simulink model "FDMA"  (Simulink 7.6)
settings: Solver=ode45  StartTime=0.0  StopTime=10.0  RelTol=1e-3
undefined symbols (not defined in the file): get, One, sided
libraries: dsparch4 x6, commanapbnd3 x6, dspsnks4 x6, commchan3 x1
settings Model: Creator=matlab  LastModifiedBy=matlab

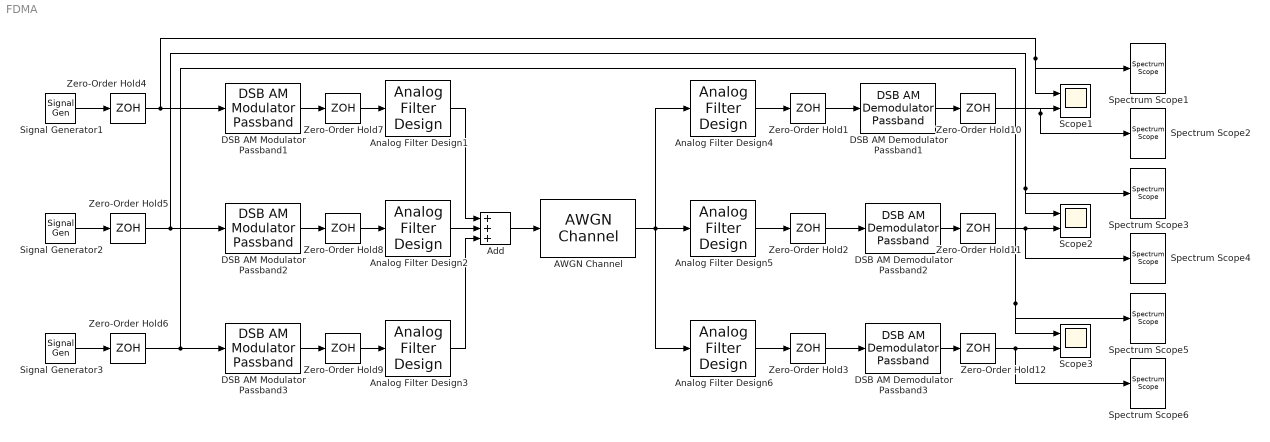
== system FDMA ==
  AWGN Channel : commchan3/AWGN Channel  SystemSampleTime=-1  InputProcessing=Columns as channels (frame based)  seed=67  noiseMode=Variance from mask  EbNodB=10  EsNodB=10  SNRdB=10  bitsPerSym=1  Ps=1  Tsym=1  variance=0.01
  Add : Sum  Inputs=+++
  Analog Filter Design1 : dsparch4/Analog Filter Design  method=Butterworth  filttype=Bandpass  N=8  Wlo=35*2*pi  Whi=45*2*pi  Rp=2  Rs=40
  Analog Filter Design2 : dsparch4/Analog Filter Design  method=Butterworth  filttype=Bandpass  N=8  Wlo=55*2*pi  Whi=65*2*pi  Rp=2  Rs=40
  Analog Filter Design3 : dsparch4/Analog Filter Design  method=Butterworth  filttype=Bandpass  N=8  Wlo=75*2*pi  Whi=85*2*pi  Rp=2  Rs=40
  Analog Filter Design4 : dsparch4/Analog Filter Design  method=Butterworth  filttype=Bandpass  N=8  Wlo=35*2*pi  Whi=45*2*pi  Rp=2  Rs=40
  Analog Filter Design5 : dsparch4/Analog Filter Design  method=Butterworth  filttype=Bandpass  N=8  Wlo=55*2*pi  Whi=65*2*pi  Rp=2  Rs=40
  Analog Filter Design6 : dsparch4/Analog Filter Design  method=Butterworth  filttype=Bandpass  N=8  Wlo=75*2*pi  Whi=85*2*pi  Rp=2  Rs=40
  DSB AM Demodulator Passband1 : commanapbnd3/DSB AM Demodulator Passband  SystemSampleTime=-1  Fc=40  Ph=0  method=Butterworth  n=4  cf=20  Rp=0.1  Rs=50  Offset=1
  DSB AM Demodulator Passband2 : commanapbnd3/DSB AM Demodulator Passband  SystemSampleTime=-1  Fc=60  Ph=0  method=Butterworth  n=4  cf=20  Rp=0.1  Rs=50  Offset=1
  DSB AM Demodulator Passband3 : commanapbnd3/DSB AM Demodulator Passband  SystemSampleTime=-1  Fc=80  Ph=0  method=Butterworth  n=4  cf=20  Rp=0.1  Rs=50  Offset=1
  DSB AM Modulator Passband1 : commanapbnd3/DSB AM Modulator Passband  SystemSampleTime=-1  Fc=40  Ph=0  Offset=1
  DSB AM Modulator Passband2 : commanapbnd3/DSB AM Modulator Passband  SystemSampleTime=-1  Fc=60  Ph=0  Offset=1
  DSB AM Modulator Passband3 : commanapbnd3/DSB AM Modulator Passband  SystemSampleTime=-1  Fc=80  Ph=0  Offset=1
  Scope1 : Scope  NumInputPorts=2
      settings: YMin=-5~-5  YMax=5~5  SampleInput=on  SampleTime=0.01
  Scope2 : Scope  NumInputPorts=2
      settings: YMin=-5~-5  YMax=5~5  SaveName=ScopeData2  SampleInput=on  SampleTime=0.01
  Scope3 : Scope  NumInputPorts=2
      settings: YMin=-5~-5  YMax=5~5  SampleInput=on  SampleTime=0.01
  Signal Generator1 : SignalGenerator  Frequency=4
  Signal Generator2 : SignalGenerator  WaveForm=square  Frequency=0.5
  Signal Generator3 : SignalGenerator  WaveForm=sawtooth
  Spectrum Scope1 : dspsnks4/Spectrum Scope  DialogController=dspdialog.SpectrumScope  DialogControllerArgs=DataTag1  SystemSampleTime=-1  ScopeProperties=on  Domain=Frequency  HorizSpan=1  UseBuffer=on  BufferSize=512  Overlap=256  inpFftLenInherit=on  FFTlength=4096  numAvg=16  DisplayProperties=off  AxisGrid=on  Memory=off  FrameNumber=on  AxisLegend=off  AxisZoom=off  OpenScopeAtSimStart=on  OpenScopeImmediately=off  FigPos=get(0,'defaultfigureposition')  AxisProperties=off  XUnits=Hertz  XRange=One-sided ([0...Fs/2])  XDisplay=0  InheritXIncr=off  XIncr=0.001  XLabel=Samples  XLimit=Auto  YUnits=Watts/Hertz  XMax=1  XMin=0  YLabel=Magnitude-squared, dB  LineProperties=off  wintypeSpecScope=Hann  RsSpecScope=50  betaSpecScope=5  winsampSpecScope=Periodic  XAxisParamsVer=6.9
      settings: YMin=0  YMax=0.40238
  Spectrum Scope2 : dspsnks4/Spectrum Scope  DialogController=dspdialog.SpectrumScope  DialogControllerArgs=DataTag2  SystemSampleTime=-1  ScopeProperties=on  Domain=Frequency  HorizSpan=1  UseBuffer=on  BufferSize=512  Overlap=256  inpFftLenInherit=on  FFTlength=4096  numAvg=16  DisplayProperties=off  AxisGrid=on  Memory=off  FrameNumber=on  AxisLegend=off  AxisZoom=off  OpenScopeAtSimStart=on  OpenScopeImmediately=off  FigPos=get(0,'defaultfigureposition')  AxisProperties=off  XUnits=Hertz  XRange=One-sided ([0...Fs/2])  XDisplay=0  InheritXIncr=off  XIncr=0.001  XLabel=Samples  XLimit=Auto  YUnits=Watts/Hertz  XMax=1  XMin=0  YLabel=Magnitude-squared, dB  LineProperties=off  wintypeSpecScope=Hann  RsSpecScope=50  betaSpecScope=5  winsampSpecScope=Periodic  XAxisParamsVer=6.9
      settings: YMin=0  YMax=0.40238
  Spectrum Scope3 : dspsnks4/Spectrum Scope  DialogController=dspdialog.SpectrumScope  DialogControllerArgs=DataTag3  SystemSampleTime=-1  ScopeProperties=on  Domain=Frequency  HorizSpan=1  UseBuffer=on  BufferSize=512  Overlap=256  inpFftLenInherit=on  FFTlength=4096  numAvg=16  DisplayProperties=off  AxisGrid=on  Memory=off  FrameNumber=on  AxisLegend=off  AxisZoom=off  OpenScopeAtSimStart=on  OpenScopeImmediately=off  FigPos=get(0,'defaultfigureposition')  AxisProperties=off  XUnits=Hertz  XRange=One-sided ([0...Fs/2])  XDisplay=0  InheritXIncr=off  XIncr=0.001  XLabel=Samples  XLimit=Auto  YUnits=Watts/Hertz  XMax=1  XMin=0  YLabel=Magnitude-squared, dB  LineProperties=off  wintypeSpecScope=Hann  RsSpecScope=50  betaSpecScope=5  winsampSpecScope=Periodic  XAxisParamsVer=6.9
      settings: YMin=0  YMax=0.40238
  Spectrum Scope4 : dspsnks4/Spectrum Scope  DialogController=dspdialog.SpectrumScope  DialogControllerArgs=DataTag4  SystemSampleTime=-1  ScopeProperties=on  Domain=Frequency  HorizSpan=1  UseBuffer=on  BufferSize=512  Overlap=256  inpFftLenInherit=on  FFTlength=4096  numAvg=16  DisplayProperties=off  AxisGrid=on  Memory=off  FrameNumber=on  AxisLegend=off  AxisZoom=off  OpenScopeAtSimStart=on  OpenScopeImmediately=off  FigPos=get(0,'defaultfigureposition')  AxisProperties=off  XUnits=Hertz  XRange=One-sided ([0...Fs/2])  XDisplay=0  InheritXIncr=off  XIncr=0.001  XLabel=Samples  XLimit=Auto  YUnits=Watts/Hertz  XMax=1  XMin=0  YLabel=Magnitude-squared, dB  LineProperties=off  wintypeSpecScope=Hann  RsSpecScope=50  betaSpecScope=5  winsampSpecScope=Periodic  XAxisParamsVer=6.9
      settings: YMin=0  YMax=0.40238
  Spectrum Scope5 : dspsnks4/Spectrum Scope  DialogController=dspdialog.SpectrumScope  DialogControllerArgs=DataTag5  SystemSampleTime=-1  ScopeProperties=on  Domain=Frequency  HorizSpan=1  UseBuffer=on  BufferSize=512  Overlap=256  inpFftLenInherit=on  FFTlength=4096  numAvg=16  DisplayProperties=off  AxisGrid=on  Memory=off  FrameNumber=on  AxisLegend=off  AxisZoom=off  OpenScopeAtSimStart=on  OpenScopeImmediately=off  FigPos=get(0,'defaultfigureposition')  AxisProperties=off  XUnits=Hertz  XRange=One-sided ([0...Fs/2])  XDisplay=0  InheritXIncr=off  XIncr=0.001  XLabel=Samples  XLimit=Auto  YUnits=Watts/Hertz  XMax=1  XMin=0  YLabel=Magnitude-squared, dB  LineProperties=off  wintypeSpecScope=Hann  RsSpecScope=50  betaSpecScope=5  winsampSpecScope=Periodic  XAxisParamsVer=6.9
      settings: YMin=0  YMax=0.40238
  Spectrum Scope6 : dspsnks4/Spectrum Scope  DialogController=dspdialog.SpectrumScope  DialogControllerArgs=DataTag6  SystemSampleTime=-1  ScopeProperties=on  Domain=Frequency  HorizSpan=1  UseBuffer=on  BufferSize=512  Overlap=256  inpFftLenInherit=on  FFTlength=4096  numAvg=16  DisplayProperties=off  AxisGrid=on  Memory=off  FrameNumber=on  AxisLegend=off  AxisZoom=off  OpenScopeAtSimStart=on  OpenScopeImmediately=off  FigPos=get(0,'defaultfigureposition')  AxisProperties=off  XUnits=Hertz  XRange=One-sided ([0...Fs/2])  XDisplay=0  InheritXIncr=off  XIncr=0.001  XLabel=Samples  XLimit=Auto  YUnits=Watts/Hertz  XMax=1  XMin=0  YLabel=Magnitude-squared, dB  LineProperties=off  wintypeSpecScope=Hann  RsSpecScope=50  betaSpecScope=5  winsampSpecScope=Periodic  XAxisParamsVer=6.9
      settings: YMin=0  YMax=0.40238
  Zero-Order Hold{1..12} (12 alike) : ZeroOrderHold  SampleTime=0.001
  wires:
  Analog Filter Design2/1 -> Add/2
  Signal Generator1/1 -> Zero-Order Hold4/1
  Signal Generator2/1 -> Zero-Order Hold5/1
  Signal Generator3/1 -> Zero-Order Hold6/1
  DSB AM Modulator Passband1/1 -> Zero-Order Hold7/1
  DSB AM Modulator Passband2/1 -> Zero-Order Hold8/1
  DSB AM Modulator Passband3/1 -> Zero-Order Hold9/1
  Analog Filter Design1/1 -> Add/1
  Analog Filter Design3/1 -> Add/3
  Add/1 -> AWGN Channel/1
  AWGN Channel/1 -> Analog Filter Design5/1, Analog Filter Design4/1, Analog Filter Design6/1
  Analog Filter Design4/1 -> Zero-Order Hold1/1
  Analog Filter Design5/1 -> Zero-Order Hold2/1
  Analog Filter Design6/1 -> Zero-Order Hold3/1
  Zero-Order Hold1/1 -> DSB AM Demodulator Passband1/1
  Zero-Order Hold2/1 -> DSB AM Demodulator Passband2/1
  Zero-Order Hold3/1 -> DSB AM Demodulator Passband3/1
  DSB AM Demodulator Passband1/1 -> Zero-Order Hold10/1
  DSB AM Demodulator Passband2/1 -> Zero-Order Hold11/1
  Zero-Order Hold4/1 -> DSB AM Modulator Passband1/1, Spectrum Scope1/1, Scope1/1
  Zero-Order Hold5/1 -> DSB AM Modulator Passband2/1, Scope2/1, Spectrum Scope3/1
  Zero-Order Hold6/1 -> DSB AM Modulator Passband3/1, Scope3/1, Spectrum Scope5/1
  Zero-Order Hold7/1 -> Analog Filter Design1/1
  Zero-Order Hold8/1 -> Analog Filter Design2/1
  Zero-Order Hold9/1 -> Analog Filter Design3/1
  Zero-Order Hold10/1 -> Spectrum Scope2/1, Scope1/2
  Zero-Order Hold11/1 -> Scope2/2, Spectrum Scope4/1
  DSB AM Demodulator Passband3/1 -> Zero-Order Hold12/1
  Zero-Order Hold12/1 -> Scope3/2, Spectrum Scope6/1
